simulink model "SSB_Net"  (R2021a)
settings: Solver=VariableStepAuto  StartTime=0.0  StopTime=10.0  RelTol=1e-3
settings Model: Creator=Bharat Gunhalkar  LastModifiedBy=Bharat Gunhalkar

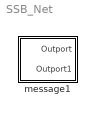
== system SSB_Net ==
  message1 : Subsystem

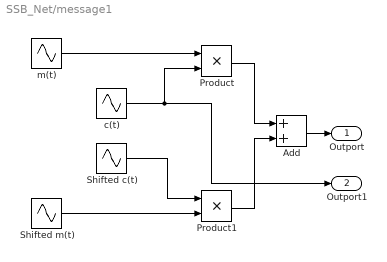
== system SSB_Net/message1 ==
  Add : Sum
  Product : Product
  Product1 : Product
  Shifted c(t) : Sin  Frequency=2*pi*1000  Phase=-(pi/2)  SampleTime=0
  Shifted m(t) : Sin  Frequency=2*pi*100  Phase=-(pi/2)  SampleTime=0
  c(t) : Sin  Frequency=2*pi*1000  SampleTime=0
  m(t) : Sin  Frequency=2*pi*100  SampleTime=0
  Outport : Outport
  Outport1 : Outport  Port=2
  wires:
  c(t)/1 -> Outport1/1, Product/2
  Shifted c(t)/1 -> Product1/1
  Shifted m(t)/1 -> Product1/2
  Product1/1 -> Add/2
  m(t)/1 -> Product/1
  Product/1 -> Add/1
  Add/1 -> Outport/1
